simulink model "quad_ndi_haller"  (R2017b)
settings: Solver=FixedStepDiscrete  StartTime=0.0  StopTime=10  FixedStep=0.004  RelTol=1e-3
libraries: simulink x5
settings Model: Creator=marcell  LastModifiedBy=Benjamin
settings DataIOCC: LimitDataPoints=on
settings OptimizationCC: DefaultParameterBehavior=Inlined  UseFloatMulNetSlope=on  DefaultUnderspecifiedDataType=single  InlineInvariantSignals=on  PassReuseOutputArgsAs=Individual arguments  ZeroExternalMemoryAtStartup=off  ZeroInternalMemoryAtStartup=off  NoFixptDivByZeroProtection=on  EfficientFloat2IntCast=on  LifeSpan=1
settings DebuggingCC: AllowSymbolicDim=off  SFUnexpectedBacktrackingDiag=warning  SFNoUnconditionalDefaultTransitionDiag=warning  SFExecutionAtInitializationDiag=none
settings HardwareCC: ProdBitPerPointer=32  ProdBitPerSizeT=32  ProdBitPerPtrDiffT=32  ProdLargestAtomicInteger=Long  ProdLargestAtomicFloat=Double  ProdWordSize=32  ProdHWDeviceType=ARM Compatible->ARM Cortex
settings ModelReferenceCC: PropagateSignalLabelsOutOfModel=off
settings SFSimCC: MATLABDynamicMemAlloc=off
settings RTWCC: SystemTargetFile=ert.tlc  GenCodeOnly=on  TemplateMakefile=ert_default_tmf  IncludeHyperlinkInReport=on  TargetLang=C++
settings CodeAppCC: ForceParamTrailComments=on  IgnoreCustomStorageClasses=off  SimulinkDataObjDesc=on  CustomSymbolStrGlobalVar=rt$N$M  CustomSymbolStrType=$N$M  CustomSymbolStrFcn=$N$M$F  CustomSymbolStrMacro=$N$M  InsertBlockDesc=on  StateflowObjectComments=on
settings ERTTargetCC: MultiwordLength=2048  GenerateSampleERTMain=on  IncludeMdlTerminateFcn=off  CombineSignalStateStructs=on  SupportAbsoluteTime=off  MultiInstanceERTCode=on  CodeInterfacePackaging=C++ class  SupportNonFinite=off  SupportComplex=off  SupportNonInlinedSFcns=on  InlinedParameterPlacement=NonHierarchical  RootIOFormat=Structure reference  ERTCustomFileTemplate=example_file_process.tlc  ERTFilePackagingFormat=CompactWithDataFile  ConvertIfToSwitch=off  SuppressUnreachableDefaultCases=off
settings ConfigComp: CovMetricSettings=dw  CovHtmlReporting=on  CovSaveCumulativeToWorkspaceVar=on  CovSaveSingleToWorkspaceVar=on  CovExternalEMLEnable=off

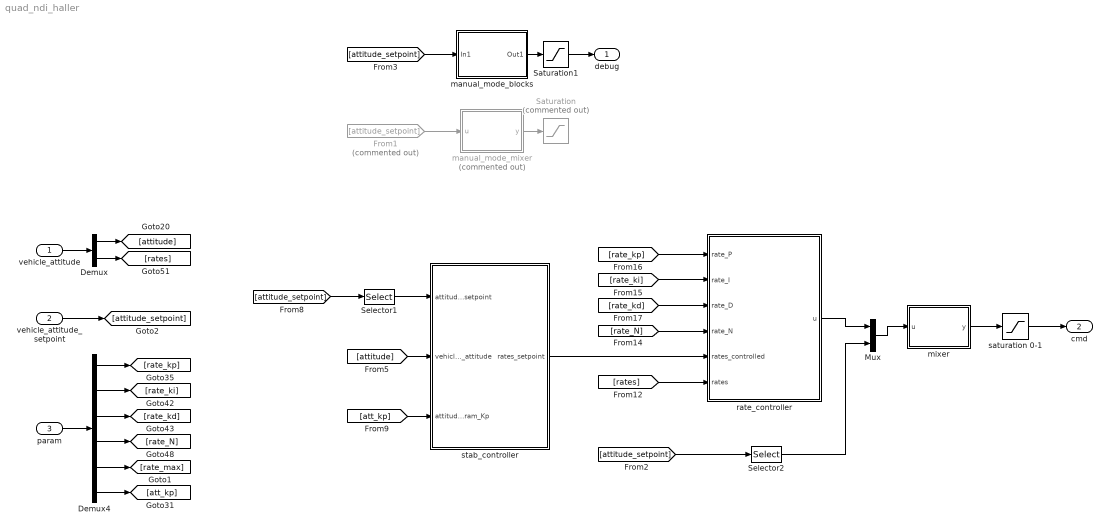
== system quad_ndi_haller ==
  vehicle_attitude : Inport  OutDataTypeStr=single  PortDimensions=6
  vehicle_attitude_setpoint : Inport  Port=2  OutDataTypeStr=single  PortDimensions=4
  param : Inport  Port=3  OutDataTypeStr=single  PortDimensions=18
  Demux : Demux  Outputs=[3 3]
  Demux4 : Demux  Outputs=[3 3 3 3 3 3]
  From1 : From  Commented=on  GotoTag=attitude_setpoint
  Mux : Mux  Inputs=2
  Saturation : Saturate  Commented=on  UpperLimit=1  LowerLimit=0  OutDataTypeStr=single
  Saturation1 : Saturate  UpperLimit=1  LowerLimit=0
  Selector1 : Selector  InputPortWidth=4  IndexOptions=Index vector (dialog)  Indices=1:3  OutputSizes=1
  Selector2 : Selector  InputPortWidth=4  IndexOptions=Index vector (dialog)  Indices=4  OutputSizes=1
  manual_mode_blocks : Subsystem
  manual_mode_mixer : MATLAB Function  Commented=on  TreatAsAtomicUnit=on
  mixer : MATLAB Function  TreatAsAtomicUnit=on
  rate_controller : Subsystem
  saturation 0-1 : Saturate  UpperLimit=1  LowerLimit=0  OutDataTypeStr=single
  stab_controller : Subsystem  TreatAsAtomicUnit=on
  debug : Outport  OutDataTypeStr=single  PortDimensions=4
  cmd : Outport  Port=2
  wires:
  vehicle_attitude/1 -> Demux/1
  Demux/1 -> [attitude]
  Demux4/1 -> [rate_kp]
  Demux4/2 -> [rate_ki]
  Demux4/3 -> [rate_kd]
  Demux4/4 -> [rate_N]
  param/1 -> Demux4/1
  Demux4/5 -> [rate_max]
  Demux4/6 -> [att_kp]
  Demux/2 -> [rates]
  vehicle_attitude_setpoint/1 -> [attitude_setpoint]
  From1/1 -> manual_mode_mixer/1(u)
  [attitude_setpoint] -> manual_mode_blocks/1(In1)
  manual_mode_blocks/1(Out1) -> Saturation1/1
  manual_mode_mixer/1(y) -> Saturation/1
  Saturation1/1 -> debug/1
  mixer/1(y) -> saturation 0-1/1
  [rate_kp] -> rate_controller/1(rate_P)
  [rate_ki] -> rate_controller/2(rate_I)
  [rate_kd] -> rate_controller/3(rate_D)
  [rate_N] -> rate_controller/4(rate_N)
  [rates] -> rate_controller/6(rates)
  saturation 0-1/1 -> cmd/1
  [att_kp] -> stab_controller/3(attitude_param_Kp)
  [attitude_setpoint] -> Selector1/1
  [attitude] -> stab_controller/2(vehicle_attitude)
  Selector1/1 -> stab_controller/1(attitude_setpoint)
  stab_controller/1(rates_setpoint) -> rate_controller/5(rates_controlled)
  rate_controller/1(u) -> Mux/1
  [attitude_setpoint] -> Selector2/1
  Selector2/1 -> Mux/2
  Mux/1 -> mixer/1(u)

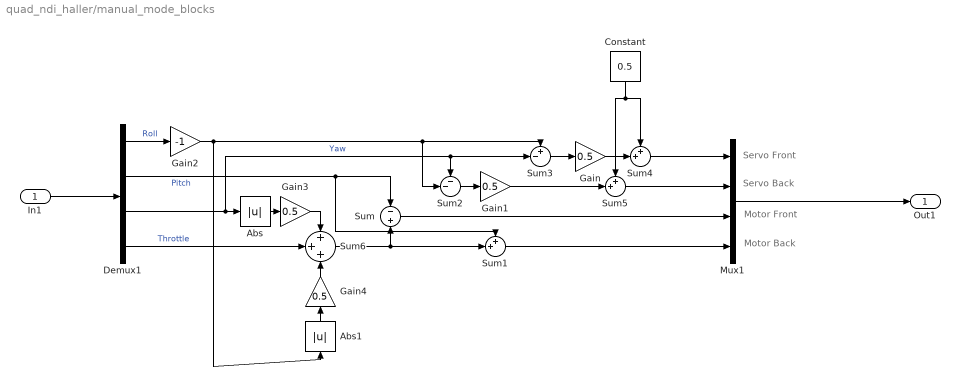
== system quad_ndi_haller/manual_mode_blocks ==
  note: Motor Back
  note: Motor Front
  note: Servo Back
  note: Servo Front
  In1 : Inport
  Abs : Abs  OutDataTypeStr=single
  Abs1 : Abs  OutDataTypeStr=single
  Constant : Constant  Value=0.5  OutDataTypeStr=single
  Demux1 : Demux
  Gain{,1,3..4} (4 alike) : Gain  Gain=0.5  OutDataTypeStr=single
  Gain2 : Gain  Gain=-1  OutDataTypeStr=single
  Mux1 : Mux
  Sum : Sum  Inputs=-+
  Sum1 : Sum  Inputs=++|
  Sum2 : Sum  Inputs=--|
  Sum3 : Sum  Inputs=+-|
  Sum4 : Sum  Inputs=++|
  Sum5 : Sum  Inputs=++|
  Sum6 : Sum  Inputs=+++
  Out1 : Outport
  wires:
  Demux1/2 -> Sum1/1, Sum/1  "Pitch"
  Sum1/1 -> Mux1/4
  Demux1/1 -> Gain2/1  "Roll"
  Sum/1 -> Mux1/3
  In1/1 -> Demux1/1
  Demux1/3 -> Sum3/2, Sum2/1, Abs/1  "Yaw"
  Constant/1 -> Sum4/1, Sum5/1
  Gain/1 -> Sum4/2
  Sum3/1 -> Gain/1
  Sum2/1 -> Gain1/1
  Gain1/1 -> Sum5/2
  Sum5/1 -> Mux1/2
  Mux1/1 -> Out1/1
  Sum4/1 -> Mux1/1
  Gain2/1 -> Abs1/1, Sum3/1, Sum2/2
  Abs/1 -> Gain3/1
  Gain3/1 -> Sum6/1
  Sum6/1 -> Sum1/2, Sum/2
  Abs1/1 -> Gain4/1
  Gain4/1 -> Sum6/3
  Demux1/4 -> Sum6/2  "Throttle"

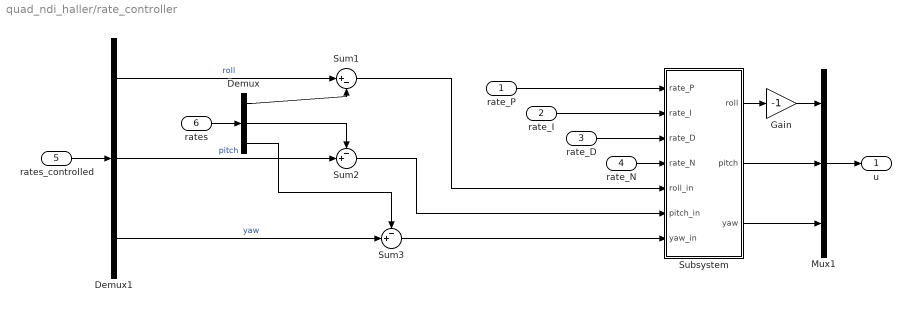
== system quad_ndi_haller/rate_controller ==
  rate_P : Inport
  rate_I : Inport  Port=2
  rate_D : Inport  Port=3
  rate_N : Inport  Port=4
  rates_controlled : Inport  Port=5
  rates : Inport  Port=6
  Demux : Demux  Outputs=3
  Demux1 : Demux  Outputs=3
  Gain : Gain  Gain=-1
  Mux1 : Mux  Inputs=3
  Subsystem : Subsystem
  Sum1 : Sum  Inputs=|+-
  Sum2 : Sum  Inputs=-+|
  Sum3 : Sum  Inputs=-+|
  u : Outport
  wires:
  Mux1/1 -> u/1
  Demux1/3 -> Sum3/2  "yaw"
  Demux1/2 -> Sum2/2  "pitch"
  rates_controlled/1 -> Demux1/1
  Demux1/1 -> Sum1/1  "roll"
  rate_P/1 -> Subsystem/1(rate_P)
  rate_I/1 -> Subsystem/2(rate_I)
  rate_D/1 -> Subsystem/3(rate_D)
  rate_N/1 -> Subsystem/4(rate_N)
  Sum1/1 -> Subsystem/5(roll_in)
  Sum2/1 -> Subsystem/6(pitch_in)
  Sum3/1 -> Subsystem/7(yaw_in)
  Subsystem/3(yaw) -> Mux1/3
  Demux/2 -> Sum2/1
  rates/1 -> Demux/1
  Subsystem/1(roll) -> Gain/1
  Subsystem/2(pitch) -> Mux1/2
  Demux/1 -> Sum1/2
  Demux/3 -> Sum3/1
  Gain/1 -> Mux1/1

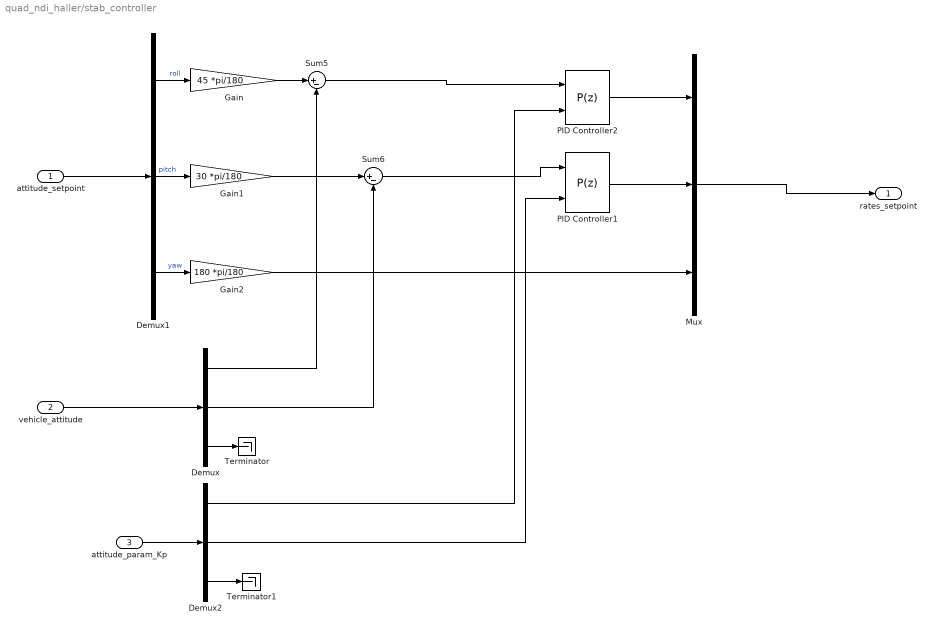
== system quad_ndi_haller/stab_controller ==
  attitude_setpoint : Inport
  vehicle_attitude : Inport  Port=2
  attitude_param_Kp : Inport  Port=3
  Demux : Demux  Outputs=3
  Demux1 : Demux  Outputs=3
  Demux2 : Demux  Outputs=3
  Gain : Gain  Gain=45 *pi/180
  Gain1 : Gain  Gain=30 *pi/180
  Gain2 : Gain  Gain=180 *pi/180
  Mux : Mux  Inputs=3
  PID Controller1 : simulink/Continuous/PID Controller  Controller=P  TimeDomain=Discrete-time  SampleTime=-1  IntegratorMethod=Forward Euler  FilterMethod=Forward Euler  Form=Parallel  UseFilter=on  ControllerParametersSource=external  P=1/0.3  I=0  D=0  N=100  InitialConditionSource=internal  InitialConditionForIntegrator=0  InitialConditionForFilter=0  ExternalReset=none  LimitOutput=off  UpperSaturationLimit=inf  LowerSaturationLimit=-inf  LinearizeAsGain=on  AntiWindupMode=none  Kb=1  TrackingMode=off  Kt=1  PParamMin=[]  PParamMax=[]  PParamDataTypeStr=single  IParamMin=[]  IParamMax=[]  IParamDataTypeStr=single  DParamMin=[]  DParamMax=[]  NParamMin=[]  NParamMax=[]  KbParamMin=[]  KbParamMax=[]  KtParamMin=[]  KtParamMax=[]  POutMin=[]  POutMax=[]  POutDataTypeStr=single  PGainOutDataTypeStr=single  PProdOutDataTypeStr=single  IOutMin=[]  IOutMax=[]  IOutDataTypeStr=single  IGainOutDataTypeStr=single  IProdOutDataTypeStr=single  DOutMin=[]  DOutMax=[]  NOutMin=[]  NOutMax=[]  KbOutMin=[]  KbOutMax=[]  KtOutMin=[]  KtOutMax=[]  IntegratorOutMin=[]  IntegratorOutMax=[]  FilterOutMin=[]  FilterOutMax=[]  SumOutMin=[]  SumOutMax=[]  SumOutDataTypeStr=single  SumI1OutMin=[]  SumI1OutMax=[]  SumI2OutMin=[]  SumI2OutMax=[]  SumI3OutMin=[]  SumI3OutMax=[]  SumDOutMin=[]  SumDOutMax=[]  SumAccumDataTypeStr=single  SaturationOutMin=[]  SaturationOutMax=[]  IntegratorContinuousStateAttributes=''  IntegratorStateMustResolveToSignalObject=off  IntegratorRTWStateStorageClass=Auto  FilterContinuousStateAttributes=''  FilterStateMustResolveToSignalObject=off  FilterRTWStateStorageClass=Auto  DifferentiatorICPrevScaledInput=0  DifferentiatorOutMin=[]  DifferentiatorOutMax=[]  InitialConditionSetting=State (most efficient)  FilterDiffOutCoefMin=[]  FilterDiffOutCoefMax=[]  SumDenOutMin=[]  SumDenOutMax=[]  SumNumOutMin=[]  SumNumOutMax=[]  ReciprocalOutMin=[]  ReciprocalOutMax=[]  DivideOutMin=[]  DivideOutMax=[]  TunerSelectOption=Transfer Function Based (PID Tuner App)
  PID Controller2 : simulink/Continuous/PID Controller  Controller=P  TimeDomain=Discrete-time  SampleTime=-1  IntegratorMethod=Forward Euler  FilterMethod=Forward Euler  Form=Parallel  UseFilter=on  ControllerParametersSource=external  P=1/0.3  I=0  D=0  N=100  InitialConditionSource=internal  InitialConditionForIntegrator=0  InitialConditionForFilter=0  ExternalReset=none  LimitOutput=off  UpperSaturationLimit=inf  LowerSaturationLimit=-inf  LinearizeAsGain=on  AntiWindupMode=none  Kb=1  TrackingMode=off  Kt=1  PParamMin=[]  PParamMax=[]  PParamDataTypeStr=single  IParamMin=[]  IParamMax=[]  IParamDataTypeStr=single  DParamMin=[]  DParamMax=[]  NParamMin=[]  NParamMax=[]  KbParamMin=[]  KbParamMax=[]  KtParamMin=[]  KtParamMax=[]  POutMin=[]  POutMax=[]  POutDataTypeStr=single  PGainOutDataTypeStr=single  PProdOutDataTypeStr=single  IOutMin=[]  IOutMax=[]  IOutDataTypeStr=single  IGainOutDataTypeStr=single  IProdOutDataTypeStr=single  DOutMin=[]  DOutMax=[]  NOutMin=[]  NOutMax=[]  KbOutMin=[]  KbOutMax=[]  KtOutMin=[]  KtOutMax=[]  IntegratorOutMin=[]  IntegratorOutMax=[]  FilterOutMin=[]  FilterOutMax=[]  SumOutMin=[]  SumOutMax=[]  SumOutDataTypeStr=single  SumI1OutMin=[]  SumI1OutMax=[]  SumI2OutMin=[]  SumI2OutMax=[]  SumI3OutMin=[]  SumI3OutMax=[]  SumDOutMin=[]  SumDOutMax=[]  SumAccumDataTypeStr=single  SaturationOutMin=[]  SaturationOutMax=[]  IntegratorContinuousStateAttributes=''  IntegratorStateMustResolveToSignalObject=off  IntegratorRTWStateStorageClass=Auto  FilterContinuousStateAttributes=''  FilterStateMustResolveToSignalObject=off  FilterRTWStateStorageClass=Auto  DifferentiatorICPrevScaledInput=0  DifferentiatorOutMin=[]  DifferentiatorOutMax=[]  InitialConditionSetting=State (most efficient)  FilterDiffOutCoefMin=[]  FilterDiffOutCoefMax=[]  SumDenOutMin=[]  SumDenOutMax=[]  SumNumOutMin=[]  SumNumOutMax=[]  ReciprocalOutMin=[]  ReciprocalOutMax=[]  DivideOutMin=[]  DivideOutMax=[]  TunerSelectOption=Transfer Function Based (PID Tuner App)
  Sum5 : Sum  Inputs=|+-
  Sum6 : Sum  Inputs=|+-
  Terminator : Terminator
  Terminator1 : Terminator
  rates_setpoint : Outport
  wires:
  Sum5/1 -> PID Controller2/1
  Sum6/1 -> PID Controller1/1
  Demux/2 -> Sum6/2
  vehicle_attitude/1 -> Demux/1
  attitude_setpoint/1 -> Demux1/1
  Demux1/1 -> Gain/1  "roll"
  Demux1/2 -> Gain1/1  "pitch"
  Demux1/3 -> Gain2/1  "yaw"
  attitude_param_Kp/1 -> Demux2/1
  Demux2/1 -> PID Controller2/2
  Demux2/2 -> PID Controller1/2
  PID Controller2/1 -> Mux/1
  PID Controller1/1 -> Mux/2
  Mux/1 -> rates_setpoint/1
  Demux/1 -> Sum5/2
  Gain2/1 -> Mux/3
  Gain/1 -> Sum5/1
  Gain1/1 -> Sum6/1
  Demux2/3 -> Terminator1/1
  Demux/3 -> Terminator/1

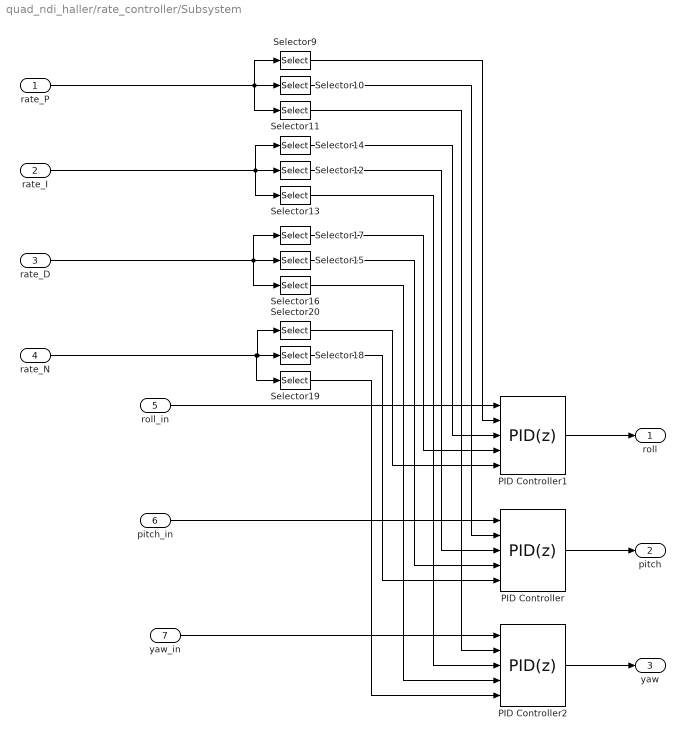
== system quad_ndi_haller/rate_controller/Subsystem ==
  rate_P : Inport
  rate_I : Inport  Port=2
  rate_D : Inport  Port=3
  rate_N : Inport  Port=4
  roll_in : Inport  Port=5
  pitch_in : Inport  Port=6
  yaw_in : Inport  Port=7
  PID Controller : simulink/Continuous/PID Controller  Controller=PID  TimeDomain=Discrete-time  SampleTime=-1  IntegratorMethod=Forward Euler  FilterMethod=Forward Euler  Form=Parallel  UseFilter=on  ControllerParametersSource=external  P=-0.119609159457863  I=-0.0298872891132111  D=-0.0962817830854201  N=11.7108788988861  InitialConditionSource=internal  InitialConditionForIntegrator=0  InitialConditionForFilter=0  ExternalReset=none  LimitOutput=off  UpperSaturationLimit=inf  LowerSaturationLimit=-inf  LinearizeAsGain=on  AntiWindupMode=none  Kb=1  TrackingMode=off  Kt=1  PParamMin=[]  PParamMax=[]  IParamMin=[]  IParamMax=[]  DParamMin=[]  DParamMax=[]  NParamMin=[]  NParamMax=[]  KbParamMin=[]  KbParamMax=[]  KtParamMin=[]  KtParamMax=[]  POutMin=[]  POutMax=[]  IOutMin=[]  IOutMax=[]  DOutMin=[]  DOutMax=[]  NOutMin=[]  NOutMax=[]  KbOutMin=[]  KbOutMax=[]  KtOutMin=[]  KtOutMax=[]  IntegratorOutMin=[]  IntegratorOutMax=[]  FilterOutMin=[]  FilterOutMax=[]  SumOutMin=[]  SumOutMax=[]  SumI1OutMin=[]  SumI1OutMax=[]  SumI2OutMin=[]  SumI2OutMax=[]  SumI3OutMin=[]  SumI3OutMax=[]  SumDOutMin=[]  SumDOutMax=[]  SaturationOutMin=[]  SaturationOutMax=[]  IntegratorContinuousStateAttributes=''  IntegratorStateMustResolveToSignalObject=off  IntegratorRTWStateStorageClass=Auto  FilterContinuousStateAttributes=''  FilterStateMustResolveToSignalObject=off  FilterRTWStateStorageClass=Auto  DifferentiatorICPrevScaledInput=0  DifferentiatorOutMin=[]  DifferentiatorOutMax=[]  InitialConditionSetting=State (most efficient)  FilterDiffOutCoefMin=[]  FilterDiffOutCoefMax=[]  SumDenOutMin=[]  SumDenOutMax=[]  SumNumOutMin=[]  SumNumOutMax=[]  ReciprocalOutMin=[]  ReciprocalOutMax=[]  DivideOutMin=[]  DivideOutMax=[]  TunerSelectOption=Transfer Function Based (PID Tuner App)
  PID Controller1 : simulink/Continuous/PID Controller  Controller=PID  TimeDomain=Discrete-time  SampleTime=-1  IntegratorMethod=Forward Euler  FilterMethod=Forward Euler  Form=Parallel  UseFilter=on  ControllerParametersSource=external  P=1  I=1  D=1  N=9.73667034237561  InitialConditionSource=internal  InitialConditionForIntegrator=0  InitialConditionForFilter=0  ExternalReset=none  LimitOutput=off  UpperSaturationLimit=inf  LowerSaturationLimit=-inf  LinearizeAsGain=on  AntiWindupMode=none  Kb=1  TrackingMode=off  Kt=1  PParamMin=[]  PParamMax=[]  PParamDataTypeStr=single  IParamMin=[]  IParamMax=[]  IParamDataTypeStr=single  DParamMin=[]  DParamMax=[]  DParamDataTypeStr=single  NParamMin=[]  NParamMax=[]  NParamDataTypeStr=single  KbParamMin=[]  KbParamMax=[]  KtParamMin=[]  KtParamMax=[]  POutMin=[]  POutMax=[]  POutDataTypeStr=single  PGainOutDataTypeStr=single  PProdOutDataTypeStr=single  IOutMin=[]  IOutMax=[]  IOutDataTypeStr=single  IGainOutDataTypeStr=single  IProdOutDataTypeStr=single  DOutMin=[]  DOutMax=[]  DOutDataTypeStr=single  DGainOutDataTypeStr=single  DProdOutDataTypeStr=single  NOutMin=[]  NOutMax=[]  NOutDataTypeStr=single  NGainOutDataTypeStr=single  NProdOutDataTypeStr=single  KbOutMin=[]  KbOutMax=[]  KtOutMin=[]  KtOutMax=[]  IntegratorOutMin=[]  IntegratorOutMax=[]  FilterOutMin=[]  FilterOutMax=[]  SumOutMin=[]  SumOutMax=[]  SumOutDataTypeStr=single  SumI1OutMin=[]  SumI1OutMax=[]  SumI2OutMin=[]  SumI2OutMax=[]  SumI3OutMin=[]  SumI3OutMax=[]  SumDOutMin=[]  SumDOutMax=[]  SumDOutDataTypeStr=single  SumAccumDataTypeStr=single  SumDAccumDataTypeStr=single  SaturationOutMin=[]  SaturationOutMax=[]  IntegratorContinuousStateAttributes=''  IntegratorStateMustResolveToSignalObject=off  IntegratorRTWStateStorageClass=Auto  FilterContinuousStateAttributes=''  FilterStateMustResolveToSignalObject=off  FilterRTWStateStorageClass=Auto  DifferentiatorICPrevScaledInput=0  DifferentiatorOutMin=[]  DifferentiatorOutMax=[]  InitialConditionSetting=State (most efficient)  FilterDiffOutCoefMin=[]  FilterDiffOutCoefMax=[]  SumDenOutMin=[]  SumDenOutMax=[]  SumNumOutMin=[]  SumNumOutMax=[]  ReciprocalOutMin=[]  ReciprocalOutMax=[]  DivideOutMin=[]  DivideOutMax=[]  TunerSelectOption=Frequency Response Based
  PID Controller2 : simulink/Continuous/PID Controller  Controller=PID  TimeDomain=Discrete-time  SampleTime=-1  IntegratorMethod=Forward Euler  FilterMethod=Forward Euler  Form=Parallel  UseFilter=on  ControllerParametersSource=external  P=0.116001216751594  I=0.0498672968614691  D=-0.0125507347856546  N=2.65016683380004  InitialConditionSource=internal  InitialConditionForIntegrator=0  InitialConditionForFilter=0  ExternalReset=none  LimitOutput=off  UpperSaturationLimit=inf  LowerSaturationLimit=-inf  LinearizeAsGain=on  AntiWindupMode=none  Kb=1  TrackingMode=off  Kt=1  PParamMin=[]  PParamMax=[]  IParamMin=[]  IParamMax=[]  DParamMin=[]  DParamMax=[]  NParamMin=[]  NParamMax=[]  KbParamMin=[]  KbParamMax=[]  KtParamMin=[]  KtParamMax=[]  POutMin=[]  POutMax=[]  IOutMin=[]  IOutMax=[]  DOutMin=[]  DOutMax=[]  NOutMin=[]  NOutMax=[]  KbOutMin=[]  KbOutMax=[]  KtOutMin=[]  KtOutMax=[]  IntegratorOutMin=[]  IntegratorOutMax=[]  FilterOutMin=[]  FilterOutMax=[]  SumOutMin=[]  SumOutMax=[]  SumI1OutMin=[]  SumI1OutMax=[]  SumI2OutMin=[]  SumI2OutMax=[]  SumI3OutMin=[]  SumI3OutMax=[]  SumDOutMin=[]  SumDOutMax=[]  SaturationOutMin=[]  SaturationOutMax=[]  IntegratorContinuousStateAttributes=''  IntegratorStateMustResolveToSignalObject=off  IntegratorRTWStateStorageClass=Auto  FilterContinuousStateAttributes=''  FilterStateMustResolveToSignalObject=off  FilterRTWStateStorageClass=Auto  DifferentiatorICPrevScaledInput=0  DifferentiatorOutMin=[]  DifferentiatorOutMax=[]  InitialConditionSetting=State (most efficient)  FilterDiffOutCoefMin=[]  FilterDiffOutCoefMax=[]  SumDenOutMin=[]  SumDenOutMax=[]  SumNumOutMin=[]  SumNumOutMax=[]  ReciprocalOutMin=[]  ReciprocalOutMax=[]  DivideOutMin=[]  DivideOutMax=[]  TunerSelectOption=Transfer Function Based (PID Tuner App)
  Selector{10,12,15,18} (4 alike) : Selector  InputPortWidth=3  IndexOptions=Index vector (dialog)  Indices=2  OutputSizes=1
  Selector{11,13,16,19} (4 alike) : Selector  InputPortWidth=3  IndexOptions=Index vector (dialog)  Indices=3  OutputSizes=1
  Selector{9,14,17,20} (4 alike) : Selector  InputPortWidth=3  IndexOptions=Index vector (dialog)  Indices=1  OutputSizes=1
  roll : Outport
  pitch : Outport  Port=2
  yaw : Outport  Port=3
  wires:
  Selector13/1 -> PID Controller2/3
  rate_I/1 -> Selector14/1, Selector12/1, Selector13/1
  Selector12/1 -> PID Controller/3
  Selector20/1 -> PID Controller1/5
  Selector15/1 -> PID Controller/4
  Selector16/1 -> PID Controller2/4
  Selector17/1 -> PID Controller1/4
  rate_D/1 -> Selector17/1, Selector16/1, Selector15/1
  Selector14/1 -> PID Controller1/3
  Selector11/1 -> PID Controller2/2
  Selector10/1 -> PID Controller/2
  rate_P/1 -> Selector9/1, Selector11/1, Selector10/1
  Selector9/1 -> PID Controller1/2
  yaw_in/1 -> PID Controller2/1
  PID Controller2/1 -> yaw/1
  pitch_in/1 -> PID Controller/1
  roll_in/1 -> PID Controller1/1
  PID Controller1/1 -> roll/1
  PID Controller/1 -> pitch/1
  rate_N/1 -> Selector19/1, Selector20/1, Selector18/1
  Selector19/1 -> PID Controller2/5
  Selector18/1 -> PID Controller/5

== matlab function quad_ndi_haller/manual_mode_mixer ==
  data: u input; y output
function y = fcn(u)

% Mixing Matrix
%     R  P  Y  T
M =  [-1  0 -1  0;  % s1
       1  0 -1  0;  % s2
       0  1  0  1;  % u1
       0 -1  0  1]; % u2

y = (M * u);

y(1) = 0.5 + 0.5 * y(1);
y(2) = 0.5 + 0.5 * y(2);
y;

== matlab function quad_ndi_haller/mixer ==
  data: u input; y output
function y = fcn(u)

% Mixing Matrix
%      R  P  Y  T
M =  [-1  0 -1  0;  % s1
       1  0 -1  0;  % s2
       0 -1  0  1;  % u1
       0  1  0  1]; % u2

% Mixing Matrix mit Steuergrößen multiplizieren   
y = M * u;

% Servo Offset, da Servocommand 0 = 90° entspricht
y(1) = 0.5 + 0.5 * y(1);
y(2) = 0.5 + 0.5 * y(2);

y;
